simulink library "Single_Track_Model_linear"  (R2018b)
settings: Solver=VariableStepAuto  StartTime=0.0  StopTime=10.0  RelTol=1e-3
undefined symbols (not defined in the file): DiscIntNeverNeededParam, par_TIR, par_VEH, psi0, psip0, v0
libraries: simulink x2, vehicle_model x1
(part 2 of 2)

== system Single_Track_Model_linear/SingleTrackModel_linear/vehicle_model/body_chassis_vert/horizontal/psipp ==
  Fls : Inport
  delta : Inport  Port=2
  F_aer : Inport  Port=3
  Bus Selector1 : BusSelector  OutputSignals=Fl.FlF,Fs.FsF,Fs.FsR
  Bus Selector2 : BusSelector  OutputSignals=F_aer_y
  Divide : Product  Inputs=*/
  Product{5,7,17,19,23,34} (6 alike) : Product  RndMeth=Zero
  Sum : Sum  Inputs=++--
  Trigonometric Function5 : Trigonometry
  Trigonometric Function6 : Trigonometry  Operator=cos
  psipp : Outport
  wires:
  Divide/1 -> psipp/1
  Sum/1 -> Divide/1
  [lDP] -> Product34/2
  Product34/1 -> Sum/4
  Bus Selector2/1 -> Product34/1  "<F_aer_y>"
  F_aer/1 -> Bus Selector2/1
  delta/1 -> Trigonometric Function6/1, Trigonometric Function5/1
  Product23/1 -> Sum/3
  Product19/1 -> Product7/2
  Trigonometric Function6/1 -> Product7/1
  Trigonometric Function5/1 -> Product5/2
  Product7/1 -> Sum/2
  Product17/1 -> Product5/1
  Product5/1 -> Sum/1
  Bus Selector1/2 -> Product19/2  "<FsF>"
  Bus Selector1/1 -> Product17/1  "<FlF>"
  Bus Selector1/3 -> Product23/1  "<FsR>"
  Fls/1 -> Bus Selector1/1
  [I_z] -> Divide/2
  [lF] -> Product19/1, Product17/2
  [lR] -> Product23/2

== system Single_Track_Model_linear/SingleTrackModel_linear/vehicle_model/body_chassis_vert/horizontal/xy_kos ==
  dv : Inport
  v : Inport  Port=2
  beta : Inport  Port=3
  betap : Inport  Port=4
  psip : Inport  Port=5
  Product{,1..6} (7 alike) : Product  RndMeth=Zero
  Sum : Sum
  Sum1 : Sum  Inputs=-+
  Sum2 : Sum
  Trigonometric Function : Trigonometry  Operator=cos
  Trigonometric Function1 : Trigonometry
  ax : Outport
  ay : Outport  Port=2
  vx : Outport  Port=3
  vy : Outport  Port=4
  wires:
  Sum2/1 -> ay/1  "ay"
  Sum1/1 -> ax/1  "ax"
  Product/1 -> Sum2/1
  Product4/1 -> Sum2/2
  Product3/1 -> Sum1/1
  Product2/1 -> Sum1/2
  Product1/1 -> Product4/2, Product3/1
  Trigonometric Function1/1 -> Product3/2, Product/1, Product6/1
  Trigonometric Function/1 -> Product4/1, Product5/1, Product2/2
  dv/1 -> Product2/1, Product/2
  v/1 -> Product6/2, Product5/2, Product1/2
  Sum/1 -> Product1/1
  betap/1 -> Sum/1
  psip/1 -> Sum/2
  beta/1 -> Trigonometric Function1/1, Trigonometric Function/1
  Product6/1 -> vy/1  "vy"
  Product5/1 -> vx/1  "vx"

== system Single_Track_Model_linear/SingleTrackModel_linear/vehicle_model/wheel/Tire Model/F ==
  Fz : Inport
  M_brems : Inport  Port=2
  M_antr : Inport  Port=3
  delta : Inport  Port=4
  beta : Inport  Port=5
  psip : Inport  Port=6
  vabs : Inport  Port=7
  TIR_parameter : Inport  Port=8
  Bus Selector1 : BusSelector  OutputSignals=UNLOADED_RADIUS
  Saturation : Saturate  UpperLimit=99999999  LowerLimit=0.001
  calc_ALPHA : Subsystem
  calc_Fx_f : Subsystem
  calc_Fy_f : Subsystem
  calc_My/M_reib : Subsystem
  calc_radius : Subsystem
  Fx : Outport
  Fy : Outport  Port=2
  My : Outport  Port=3
  alpha : Outport  Port=4
  r_dyn : Outport  Port=5
  r_stat : Outport  Port=6
  wires:
  calc_ALPHA/1(ALPHA) -> alpha/1, calc_Fy_f/1(alpha)  "alpha_F"
  Saturation/1 -> calc_My/M_reib/1(Fz)
  calc_radius/1(r_stat_F) -> r_stat/1  "r_stat_F"
  calc_radius/2(r_dyn_F) -> calc_My/M_reib/2(r_dyn), r_dyn/1, calc_Fx_f/4(r_dyn)  "r_dyn_F"
  Fz/1 -> Saturation/1
  TIR_parameter/1 -> Bus Selector1/1
  calc_My/M_reib/1(My) -> calc_Fx_f/1(M_reib), My/1  "My_f"
  M_antr/1 -> calc_Fx_f/3(M_antr)
  M_brems/1 -> calc_Fx_f/2(M_brems)
  vabs/1 -> calc_ALPHA/1(v)
  delta/1 -> calc_ALPHA/2(delta)
  beta/1 -> calc_ALPHA/3(beta)
  psip/1 -> calc_ALPHA/4(psip)
  calc_Fx_f/1(Fx_f) -> Fx/1  "FlF"
  calc_Fy_f/1(Fy_f) -> Fy/1  "FsF"
  Bus Selector1/1 -> calc_radius/1(UNLOADED_RADIUS)  "<UNLOADED_RADIUS>"

== system Single_Track_Model_linear/SingleTrackModel_linear/vehicle_model/wheel/Tire Model/R ==
  vabs : Inport
  psip : Inport  Port=2
  beta : Inport  Port=3
  Fz : Inport  Port=4
  M_brems : Inport  Port=5
  M_antr : Inport  Port=6
  TIR_parameter : Inport  Port=7
  Bus Selector1 : BusSelector  OutputSignals=UNLOADED_RADIUS
  Saturation : Saturate  UpperLimit=99999999  LowerLimit=0.001
  calc_ALPHA : Subsystem
  calc_Fx_r : Subsystem
  calc_Fy_r : Subsystem
  calc_My/M_reib : Subsystem
  calc_radius : Subsystem
  Fx : Outport
  Fy : Outport  Port=2
  My : Outport  Port=3
  alpha : Outport  Port=4
  r_dyn : Outport  Port=5
  r_stat : Outport  Port=6
  wires:
  calc_Fx_r/1(Fx_r) -> Fx/1  "FlR"
  psip/1 -> calc_ALPHA/3(psip)
  beta/1 -> calc_ALPHA/2(beta)
  vabs/1 -> calc_ALPHA/1(v)
  M_brems/1 -> calc_Fx_r/2(M_brems)
  M_antr/1 -> calc_Fx_r/3(M_antr)
  calc_My/M_reib/1(My) -> My/1, calc_Fx_r/1(M_reib)  "My_r"
  Fz/1 -> Saturation/1
  calc_radius/2(r_dyn_R) -> r_dyn/1, calc_Fx_r/4(r_dyn), calc_My/M_reib/2(r_dyn)  "r_dyn_R"
  calc_Fy_r/1(Fy_r) -> Fy/1  "FsR"
  calc_radius/1(r_stat_R) -> r_stat/1  "r_stat_R"
  Saturation/1 -> calc_My/M_reib/1(Fz)
  calc_ALPHA/1(ALPHA) -> calc_Fy_r/1(alpha), alpha/1  "alpha_R"
  TIR_parameter/1 -> Bus Selector1/1
  Bus Selector1/1 -> calc_radius/1(UNLOADED_RADIUS)  "<UNLOADED_RADIUS>"

== system Single_Track_Model_linear/SingleTrackModel_linear/vehicle_model/wheel/calc_v/calc_vl ==
  lF : Inport
  v : Inport  Port=2
  psi : Inport  Port=3
  beta : Inport  Port=4
  delta : Inport  Port=5
  Bus Creator : BusCreator  Inputs=2
  Bus Selector : BusSelector  OutputSignals=YawAngleVelocityPsip [rad/s]
  Bus Selector2 : BusSelector  OutputSignals=SideSlipAngleBeta [rad]
  Product{,1,5..7} (5 alike) : Product  RndMeth=Zero
  Subtract1 : Sum
  Subtract2 : Sum
  Trigonometric Function : Trigonometry
  Trigonometric Function1 : Trigonometry  Operator=cos
  Trigonometric Function2 : Trigonometry
  Trigonometric Function3 : Trigonometry  Operator=cos
  vl : Outport
  wires:
  Subtract1/1 -> Bus Creator/1  "vl_F"
  Product/1 -> Bus Creator/2, Product6/2  "vl_R"
  Bus Creator/1 -> vl/1
  psi/1 -> Bus Selector/1
  beta/1 -> Bus Selector2/1
  Bus Selector2/1 -> Trigonometric Function1/1, Trigonometric Function/1  "<SideSlipAngleBeta [rad]>"
  v/1 -> Product1/2, Product/1
  Trigonometric Function1/1 -> Product/2
  Trigonometric Function/1 -> Product1/1
  Bus Selector/1 -> Product5/2  "<YawAngleVelocityPsip [rad/s]>"
  lF/1 -> Product5/1
  delta/1 -> Trigonometric Function2/1, Trigonometric Function3/1
  Trigonometric Function3/1 -> Product6/1
  Product6/1 -> Subtract1/2
  Product7/1 -> Subtract1/1
  Trigonometric Function2/1 -> Product7/2
  Subtract2/1 -> Product7/1
  Product1/1 -> Subtract2/2
  Product5/1 -> Subtract2/1

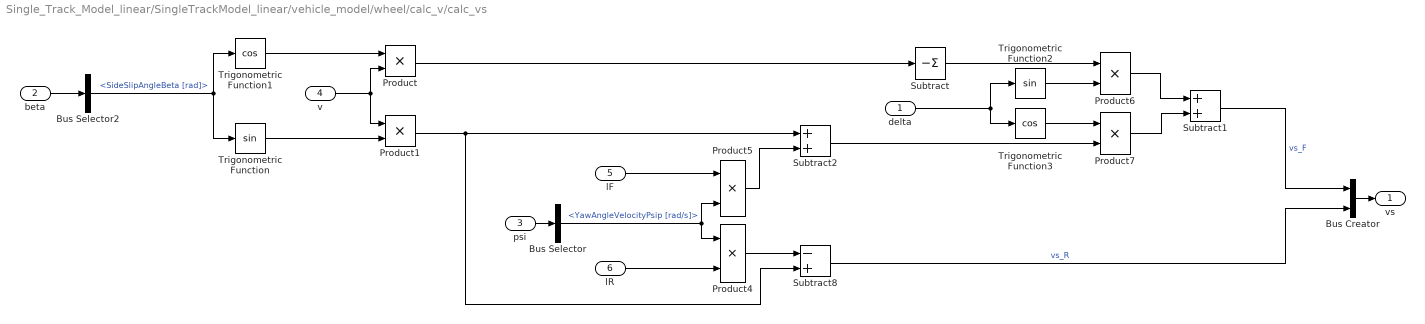
== system Single_Track_Model_linear/SingleTrackModel_linear/vehicle_model/wheel/calc_v/calc_vs ==
  delta : Inport
  beta : Inport  Port=2
  psi : Inport  Port=3
  v : Inport  Port=4
  lF : Inport  Port=5
  lR : Inport  Port=6
  Bus Creator : BusCreator  Inputs=2
  Bus Selector : BusSelector  OutputSignals=YawAngleVelocityPsip [rad/s]
  Bus Selector2 : BusSelector  OutputSignals=SideSlipAngleBeta [rad]
  Product{,1,4..7} (6 alike) : Product  RndMeth=Zero
  Subtract : Sum  Inputs=-
  Subtract1 : Sum
  Subtract2 : Sum
  Subtract8 : Sum  Inputs=-+
  Trigonometric Function : Trigonometry
  Trigonometric Function1 : Trigonometry  Operator=cos
  Trigonometric Function2 : Trigonometry
  Trigonometric Function3 : Trigonometry  Operator=cos
  vs : Outport
  wires:
  Product4/1 -> Subtract8/1
  Product5/1 -> Subtract2/2
  Product1/1 -> Subtract8/2, Subtract2/1
  Subtract2/1 -> Product7/2
  Trigonometric Function3/1 -> Product7/1
  Product7/1 -> Subtract1/2
  Product6/1 -> Subtract1/1
  Trigonometric Function2/1 -> Product6/2
  Subtract/1 -> Product6/1
  Product/1 -> Subtract/1
  delta/1 -> Trigonometric Function2/1, Trigonometric Function3/1
  lR/1 -> Product4/2
  lF/1 -> Product5/1
  Trigonometric Function/1 -> Product1/2
  Trigonometric Function1/1 -> Product/1
  v/1 -> Product1/1, Product/2
  Bus Selector2/1 -> Trigonometric Function/1, Trigonometric Function1/1  "<SideSlipAngleBeta [rad]>"
  beta/1 -> Bus Selector2/1
  psi/1 -> Bus Selector/1
  Bus Creator/1 -> vs/1
  Subtract8/1 -> Bus Creator/2  "vs_R"
  Subtract1/1 -> Bus Creator/1  "vs_F"
  Bus Selector/1 -> Product4/1, Product5/2  "<YawAngleVelocityPsip [rad/s]>"

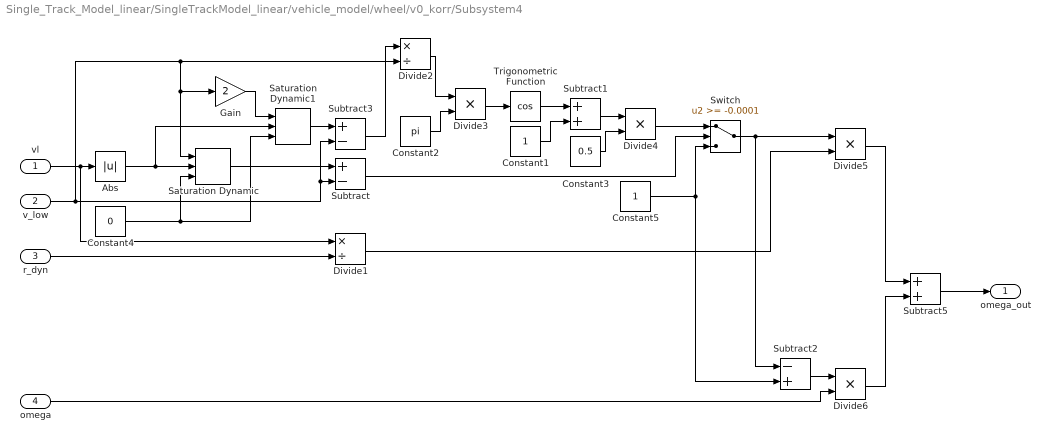
== system Single_Track_Model_linear/SingleTrackModel_linear/vehicle_model/wheel/v0_korr/Subsystem4 ==
  vl : Inport
  v_low : Inport  Port=2
  r_dyn : Inport  Port=3
  omega : Inport  Port=4
  Abs : Abs
  Constant1 : Constant
  Constant2 : Constant  Value=pi
  Constant3 : Constant  Value=0.5
  Constant4 : Constant  Value=0  VectorParams1D=off
  Constant5 : Constant
  Divide1 : Product  Inputs=*/
  Divide2 : Product  Inputs=*/
  Divide{3..6} (4 alike) : Product  Inputs=**
  Gain : Gain  Gain=2
  Saturation Dynamic : simulink/Discontinuities/Saturation Dynamic  OutMin=[]  OutMax=[]  OutDataTypeStr=Inherit: Same as second input  OutDataType=fixdt(1, 16)  OutScaling=2^-10  DoSatur=off
  Saturation Dynamic1 : simulink/Discontinuities/Saturation Dynamic  OutMin=[]  OutMax=[]  OutDataTypeStr=Inherit: Same as second input  OutDataType=fixdt(1, 16)  OutScaling=2^-10  DoSatur=off
  Subtract : Sum  Inputs=+-
  Subtract1 : Sum
  Subtract2 : Sum  Inputs=-+
  Subtract3 : Sum  Inputs=+-
  Subtract5 : Sum
  Switch : Switch  Threshold=-0.0001
  Trigonometric Function : Trigonometry  Operator=cos
  omega_out : Outport
  wires:
  Gain/1 -> Saturation Dynamic1/1
  Saturation Dynamic1/1 -> Subtract3/1
  Subtract3/1 -> Divide2/1
  Subtract2/1 -> Divide6/1
  Divide5/1 -> Subtract5/1
  Switch/1 -> Subtract2/1, Divide5/1
  Constant5/1 -> Subtract2/2, Switch/3
  Divide4/1 -> Switch/1
  Divide6/1 -> Subtract5/2
  Subtract5/1 -> omega_out/1
  omega/1 -> Divide6/2
  Constant4/1 -> Saturation Dynamic/3, Saturation Dynamic1/3
  Saturation Dynamic/1 -> Subtract/1
  Abs/1 -> Saturation Dynamic1/2, Saturation Dynamic/2
  Constant3/1 -> Divide4/2
  Subtract1/1 -> Divide4/1
  Constant1/1 -> Subtract1/2
  Trigonometric Function/1 -> Subtract1/1
  Divide3/1 -> Trigonometric Function/1
  Constant2/1 -> Divide3/2
  Divide2/1 -> Divide3/1
  Subtract/1 -> Switch/2
  r_dyn/1 -> Divide1/2
  v_low/1 -> Gain/1, Saturation Dynamic/1, Divide2/2, Subtract3/2, Subtract/2
  Divide1/1 -> Divide5/2
  vl/1 -> Divide1/1, Abs/1

== system Single_Track_Model_linear/SingleTrackModel_linear/vehicle_model/body_chassis_vert/horizontal/betap/Blending ==
  betapin : Inport
  absVx : Inport  Port=2
  Bias : Bias  Bias=1
  Bias1 : Bias  Bias=-2*pi
  Gain : Gain  Gain=2*pi*0.5
  Gain1 : Gain  Gain=0.5
  Product : Product  RndMeth=Zero
  Trigonometric Function : Trigonometry  Operator=tanh
  betapout : Outport
  wires:
  Gain1/1 -> Product/1
  Bias/1 -> Gain1/1
  Trigonometric Function/1 -> Bias/1
  Bias1/1 -> Trigonometric Function/1
  Gain/1 -> Bias1/1
  absVx/1 -> Gain/1
  Product/1 -> betapout/1
  betapin/1 -> Product/2

== system Single_Track_Model_linear/SingleTrackModel_linear/vehicle_model/wheel/Tire Model/F/calc_ALPHA ==
  v : Inport
  delta : Inport  Port=2
  beta : Inport  Port=3
  psip : Inport  Port=4
  Abs2 : Abs
  Add : Sum  Inputs=+--
  Constant1 : Constant  Value=0
  Divide1 : Product  Inputs=**/
  Switch2 : Switch  Threshold=1
  ALPHA : Outport
  wires:
  Abs2/1 -> Switch2/2
  Switch2/1 -> ALPHA/1
  Constant1/1 -> Switch2/3
  delta/1 -> Add/1
  beta/1 -> Add/2
  [lF] -> Divide1/1
  psip/1 -> Divide1/2
  Divide1/1 -> Add/3
  Add/1 -> Switch2/1
  v/1 -> Abs2/1, Divide1/3

== system Single_Track_Model_linear/SingleTrackModel_linear/vehicle_model/wheel/Tire Model/F/calc_Fx_f ==
  M_reib : Inport
  M_brems : Inport  Port=2
  M_antr : Inport  Port=3
  r_dyn : Inport  Port=4
  Divide : Product  Inputs=*/
  Sum : Sum  Inputs=+++
  Fx_f : Outport
  wires:
  Divide/1 -> Fx_f/1
  Sum/1 -> Divide/1
  M_antr/1 -> Sum/1
  M_brems/1 -> Sum/2
  M_reib/1 -> Sum/3
  r_dyn/1 -> Divide/2

== system Single_Track_Model_linear/SingleTrackModel_linear/vehicle_model/wheel/Tire Model/F/calc_Fy_f ==
  alpha : Inport
  Product : Product
  Fy_f : Outport
  wires:
  Product/1 -> Fy_f/1
  alpha/1 -> Product/2
  [c_alpha_F] -> Product/1

== system Single_Track_Model_linear/SingleTrackModel_linear/vehicle_model/wheel/Tire Model/F/calc_My//M_reib ==
  Fz : Inport
  r_dyn : Inport  Port=2
  Gain : Gain  Gain=-1
  Product : Product  Inputs=3
  crr : Constant  Value=0.012
  My : Outport
  wires:
  r_dyn/1 -> Product/2
  Fz/1 -> Product/3
  crr/1 -> Product/1
  Product/1 -> Gain/1
  Gain/1 -> My/1

== system Single_Track_Model_linear/SingleTrackModel_linear/vehicle_model/wheel/Tire Model/F/calc_radius ==
  note: r_dyn=r_stat+2/3*(r0-r_stat) [Fahrzeugdynamik - Mechanik des bewegten Fahrzeugs - Kapitel 2 (http://www.springer.com/978-3-658-09474-4)]
      |
      | r_stat~0,95*r0 [Grundlagen KFZ,Lienkamp, 6-24]
      |
      | ->r_dyn~0,95*r0+2/3*0,05*r0
      |
      | -> r_dyn~0,95*r0+1/30*r0
      |
      | -> r_dyn~59/60*r0
  UNLOADED_RADIUS : Inport
  Gain : Gain  Gain=0.95
  Gain1 : Gain  Gain=(59/60)
  r_stat_F : Outport
  r_dyn_F : Outport  Port=2
  wires:
  UNLOADED_RADIUS/1 -> Gain1/1, Gain/1
  Gain/1 -> r_stat_F/1  "r_stat_F"
  Gain1/1 -> r_dyn_F/1  "r_dyn_F"

== system Single_Track_Model_linear/SingleTrackModel_linear/vehicle_model/wheel/Tire Model/R/calc_ALPHA ==
  v : Inport
  beta : Inport  Port=2
  psip : Inport  Port=3
  Abs2 : Abs
  Add : Sum  Inputs=+-
  Constant1 : Constant  Value=0
  Divide1 : Product  Inputs=**/
  Switch2 : Switch  Threshold=1
  ALPHA : Outport
  wires:
  Abs2/1 -> Switch2/2
  Switch2/1 -> Add/1
  Constant1/1 -> Switch2/3
  v/1 -> Abs2/1, Divide1/3
  Add/1 -> ALPHA/1
  Divide1/1 -> Switch2/1
  psip/1 -> Divide1/2
  [lR] -> Divide1/1
  beta/1 -> Add/2

== system Single_Track_Model_linear/SingleTrackModel_linear/vehicle_model/wheel/Tire Model/R/calc_Fx_r ==
  M_reib : Inport
  M_brems : Inport  Port=2
  M_antr : Inport  Port=3
  r_dyn : Inport  Port=4
  Divide : Product  Inputs=*/
  Sum : Sum  Inputs=+++
  Fx_r : Outport
  wires:
  Divide/1 -> Fx_r/1
  Sum/1 -> Divide/1
  r_dyn/1 -> Divide/2
  M_reib/1 -> Sum/3
  M_brems/1 -> Sum/2
  M_antr/1 -> Sum/1

== system Single_Track_Model_linear/SingleTrackModel_linear/vehicle_model/wheel/Tire Model/R/calc_Fy_r ==
  alpha : Inport
  Product : Product
  Fy_r : Outport
  wires:
  [c_alpha_R] -> Product/1
  alpha/1 -> Product/2
  Product/1 -> Fy_r/1

== system Single_Track_Model_linear/SingleTrackModel_linear/vehicle_model/wheel/Tire Model/R/calc_My//M_reib ==
  Fz : Inport
  r_dyn : Inport  Port=2
  Gain : Gain  Gain=-1
  Product : Product  Inputs=3
  crr : Constant  Value=0.012
  My : Outport
  wires:
  Gain/1 -> My/1
  Product/1 -> Gain/1
  crr/1 -> Product/1
  Fz/1 -> Product/3
  r_dyn/1 -> Product/2

== system Single_Track_Model_linear/SingleTrackModel_linear/vehicle_model/wheel/Tire Model/R/calc_radius ==
  note: r_dyn=r_stat+2/3*(r0-r_stat) [Fahrzeugdynamik - Mechanik des bewegten Fahrzeugs - Kapitel 2 (http://www.springer.com/978-3-658-09474-4)]
      |
      | r_stat~0,95*r0 [Grundlagen KFZ,Lienkamp, 6-24]
      |
      | ->r_dyn~0,95*r0+2/3*0,05*r0
      |
      | -> r_dyn~0,95*r0+1/30*r0
      |
      | -> r_dyn~59/60*r0
  UNLOADED_RADIUS : Inport
  Gain : Gain  Gain=0.95
  Gain1 : Gain  Gain=(59/60)
  r_stat_R : Outport
  r_dyn_R : Outport  Port=2
  wires:
  UNLOADED_RADIUS/1 -> Gain1/1, Gain/1
  Gain/1 -> r_stat_R/1  "r_stat_R"
  Gain1/1 -> r_dyn_R/1  "r_dyn_R"
